simulink model "Lab1_DynamicDecoupledPlantModel_embedded"  (R2019a)
settings: Solver=VariableStepAuto  StartTime=0.0  StopTime=100  RelTol=1e-3
libraries: cstblocks x2
settings Model: Creator=emma  LastModifiedBy=emma

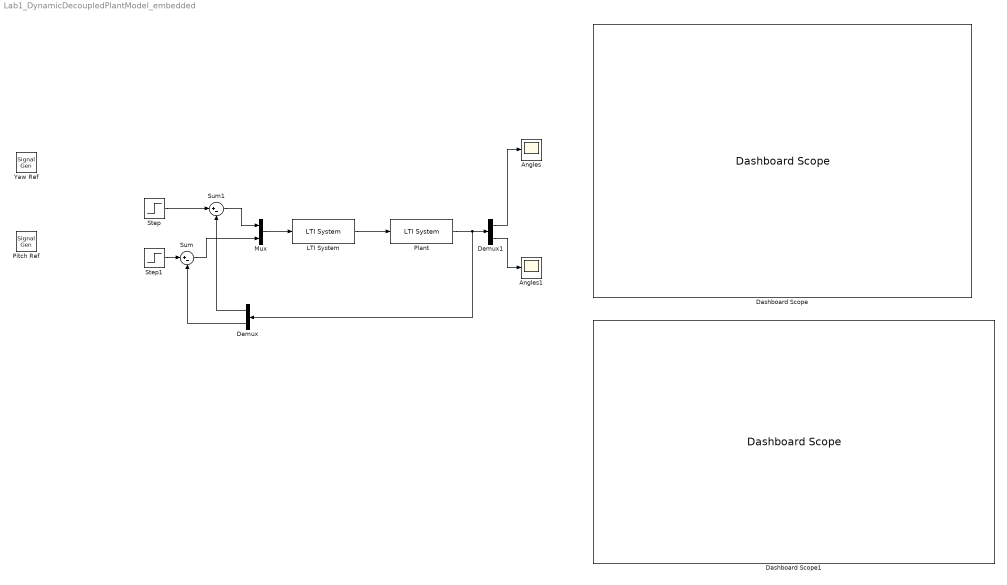
== system Lab1_DynamicDecoupledPlantModel_embedded ==
  Angles : Scope
  Angles1 : Scope
  Dashboard Scope : DashboardScope
  Dashboard Scope1 : DashboardScope
  Demux : Demux  Outputs=2
  Demux1 : Demux  Outputs=2
  LTI System : cstblocks/LTI System  sys=Kdecoupling  IC=[]
  Mux : Mux  Inputs=2
  Pitch Ref : SignalGenerator  WaveForm=square  Amplitude=pi/6  Frequency=0.4  Units=rad/sec
  Plant : cstblocks/LTI System  sys=Gnom  IC=[]
  Step : Step  SampleTime=0  VectorParams1D=off
  Step1 : Step  SampleTime=0
  Sum : Sum  Inputs=|+-
  Sum1 : Sum  Inputs=|+-
  Yaw Ref : SignalGenerator  WaveForm=square  Amplitude=pi/4  Frequency=0.5  Units=rad/sec
  wires:
  Demux/1 -> Sum1/2
  Demux/2 -> Sum/2
  Sum1/1 -> Mux/1
  Sum/1 -> Mux/2
  Step1/1 -> Sum/1
  Step/1 -> Sum1/1
  Mux/1 -> LTI System/1
  LTI System/1 -> Plant/1
  Plant/1 -> Demux/1, Demux1/1
  Demux1/1 -> Angles/1
  Demux1/2 -> Angles1/1
